simulink model "model1"  (R2022a)
settings: Solver=FixedStepAuto  StartTime=0.0  StopTime=25  FixedStep=0.0001  RelTol=1e-3
undefined symbols (not defined in the file): A, d, Jdv, kdv, kred, kyy, n, Tm, w
settings Model: Creator=max  LastModifiedBy=Family
settings SolverCC: AlgebraicLoopSolver=TrustRegion
settings DebuggingCC: UnconnectedInputMsg=warning  UnconnectedOutputMsg=warning  UnconnectedLineMsg=warning  SFMachineParentedDataDiag=warning
settings RTWCC: DLArmComputeVersion=19.05

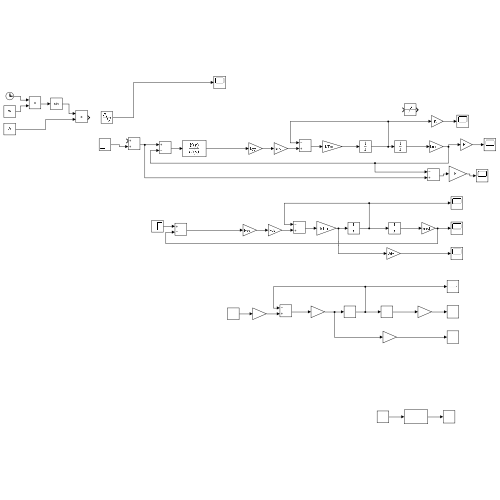
[thumbnail: Simulink's stored preview of the top-level diagram]
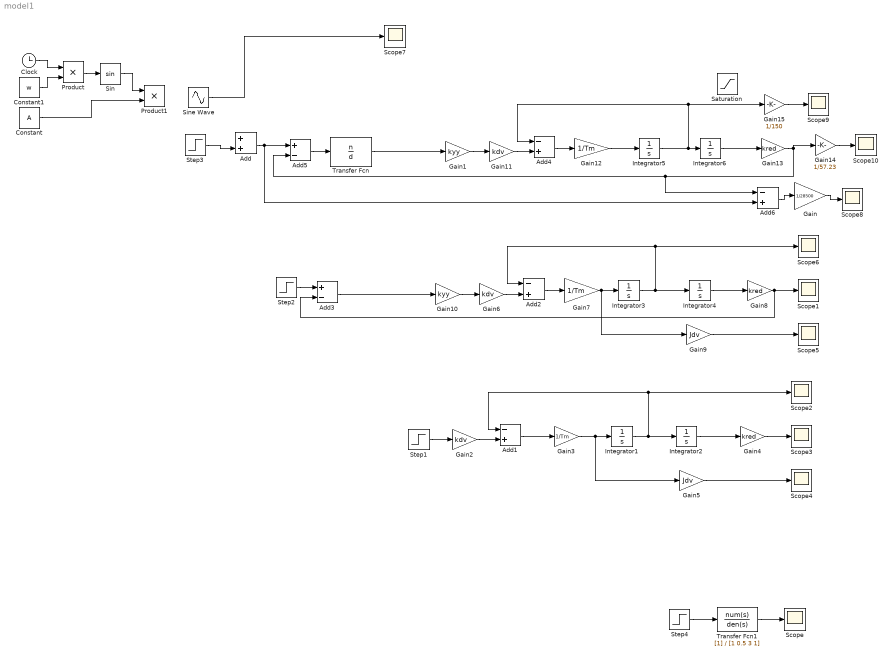
== system model1 ==
  Add : Sum
  Add{1..2,4,6} (4 alike) : Sum  Inputs=-+
  Add3 : Sum  Inputs=+-
  Add5 : Sum  Inputs=+-
  Clock : Clock
  Constant : Constant  Value=A
  Constant1 : Constant  Value=w
  Gain : Gain  Gain=1/28500
  Gain1 : Gain  Gain=kyy
  Gain10 : Gain  Gain=kyy
  Gain11 : Gain  Gain=kdv
  Gain12 : Gain  Gain=1/Tm
  Gain13 : Gain  Gain=kred
  Gain14 : Gain  Gain=1/57.23
  Gain15 : Gain  Gain=1/150
  Gain2 : Gain  Gain=kdv
  Gain3 : Gain  Gain=1/Tm
  Gain4 : Gain  Gain=kred
  Gain5 : Gain  Gain=Jdv
  Gain6 : Gain  Gain=kdv
  Gain7 : Gain  Gain=1/Tm
  Gain8 : Gain  Gain=kred
  Gain9 : Gain  Gain=Jdv
  Integrator{1..6} (6 alike) : Integrator
  Product : Product
  Product1 : Product
  Saturation : Saturate  UpperLimit=6.5  LowerLimit=-6.5
  Scope{,1..10} (11 alike) : Scope
  Sin : Trigonometry
  Sine Wave : Sin  Amplitude=A  Frequency=w  SampleTime=0
  Step1 : Step  After=45
  Step2 : Step  After=45
  Step3 : Step  Time=0  After=45
  Step4 : Step  Time=0
  Transfer Fcn : TransferFcn  Numerator=n  Denominator=d
  Transfer Fcn1 : TransferFcn  Denominator=[1 0.5 3 1]
  wires:
  Step1/1 -> Gain2/1
  Gain2/1 -> Add1/2
  Add1/1 -> Gain3/1
  Gain3/1 -> Integrator1/1, Gain5/1
  Integrator1/1 -> Integrator2/1, Add1/1, Scope2/1
  Integrator2/1 -> Gain4/1
  Gain4/1 -> Scope3/1
  Gain5/1 -> Scope4/1
  Gain6/1 -> Add2/2
  Integrator3/1 -> Integrator4/1, Scope6/1, Add2/1
  Integrator4/1 -> Gain8/1
  Gain7/1 -> Integrator3/1, Gain9/1
  Add2/1 -> Gain7/1
  Gain9/1 -> Scope5/1
  Gain8/1 -> Scope1/1, Add3/2
  Add3/1 -> Gain10/1
  Step2/1 -> Add3/1
  Gain10/1 -> Gain6/1
  Gain13/1 -> Gain14/1, Add5/2, Add6/1
  Gain11/1 -> Add4/2
  Integrator6/1 -> Gain13/1
  Add4/1 -> Gain12/1
  Integrator5/1 -> Add4/1, Gain15/1, Integrator6/1
  Gain1/1 -> Gain11/1
  Add5/1 -> Transfer Fcn/1
  Transfer Fcn/1 -> Gain1/1
  Add6/1 -> Gain/1
  Clock/1 -> Product/1
  Constant1/1 -> Product/2
  Product/1 -> Sin/1
  Sin/1 -> Product1/1
  Constant/1 -> Product1/2
  Add/1 -> Add5/1, Add6/2
  Step4/1 -> Transfer Fcn1/1
  Transfer Fcn1/1 -> Scope/1
  Gain12/1 -> Integrator5/1
  Sine Wave/1 -> Scope7/1
  Gain/1 -> Scope8/1
  Gain14/1 -> Scope10/1
  Gain15/1 -> Scope9/1
  Step3/1 -> Add/2
